simulink model "apoorva"  (R2018b)
settings: Solver=VariableStepAuto  StartTime=0  StopTime=10.0  RelTol=1e-3
values from neighbouring files (symbols this model uses):
  B = 16    [apoorvasim.m]
  k = 16    [apoorvasim.m]
  M = 2    [apoorvasim.m]
settings Model: Creator=student  LastModifiedBy=student

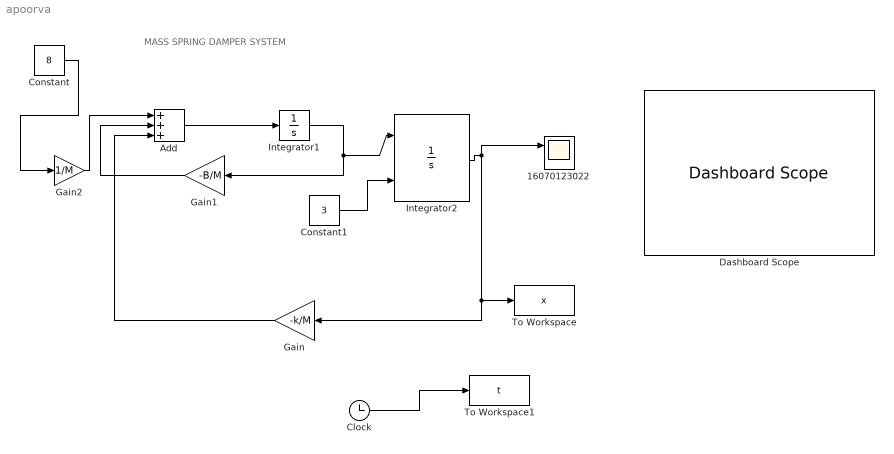
== system apoorva ==
  note: MASS SPRING DAMPER SYSTEM
  16070123022 : Scope  NumInputPorts=2
  Add : Sum  Inputs=+++
  Clock : Clock
  Constant : Constant  Value=8
  Constant1 : Constant  Value=3
  Dashboard Scope : DashboardScope  WebBlockId=8
  Gain : Gain  Gain=-k/M
  Gain1 : Gain  Gain=-B/M
  Gain2 : Gain  Gain=1/M
  Integrator1 : Integrator
  Integrator2 : Integrator  InitialConditionSource=external  InitialCondition=5
  To Workspace : ToWorkspace  VariableName=x  SampleTime=-1
  To Workspace1 : ToWorkspace  VariableName=t  SampleTime=-1
  wires:
  Integrator2/1 -> 16070123022/1, To Workspace/1, Gain/1
  Add/1 -> Integrator1/1
  Constant/1 -> Gain2/1
  Gain2/1 -> Add/1
  Gain1/1 -> Add/2
  Gain/1 -> Add/3
  Integrator1/1 -> Gain1/1, Integrator2/1
  Constant1/1 -> Integrator2/2
  Clock/1 -> To Workspace1/1
